simulink model "assignment_port_complex_test"  (Simulink 8.4)
settings: Solver=VariableStepDiscrete  StartTime=0.0  StopTime=0  MaxStep=1  RelTol=1e-3
settings Model: Creator=arnaud  LastModifiedBy=arnaud
settings DataIOCC: ExternalInput=xin  LoadExternalInput=on  SaveFormat=Structure  SignalLoggingSaveFormat=Dataset
settings OptimizationCC: ExpressionDepthLimit=128
settings DebuggingCC: UnderspecifiedInitializationDetection=Simplified  MergeDetectMultiDrivingBlocksExec=error  FcnCallInpInsideContextMsg=EnableAllAsError  StateNameClashWarn=none
settings GRTTargetCC: CombineOutputUpdateFcns=on  GRTInterface=off

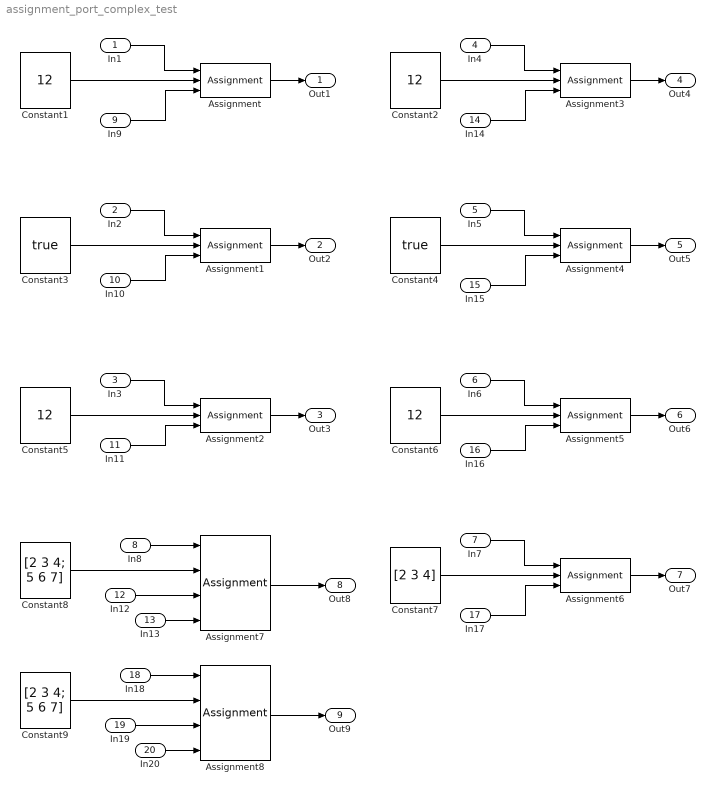
== system assignment_port_complex_test ==
  In1 : Inport  PortDimensions=[2 3]
      settings: SignalType=complex
  In2 : Inport  Port=2  OutDataTypeStr=boolean  PortDimensions=[2 3]
  In3 : Inport  Port=3  OutDataTypeStr=int32  PortDimensions=[2 3]
      settings: SignalType=complex
  In4 : Inport  Port=4  PortDimensions=3
      settings: SignalType=complex
  In5 : Inport  Port=5  OutDataTypeStr=boolean  PortDimensions=3
  In6 : Inport  Port=6  OutDataTypeStr=int32  PortDimensions=3
      settings: SignalType=complex
  In7 : Inport  Port=7  OutDataTypeStr=int32  PortDimensions=3
      settings: SignalType=complex
  In8 : Inport  Port=8  OutDataTypeStr=int32  PortDimensions=[2 3]
      settings: SignalType=complex
  In9 : Inport  Port=9  PortDimensions=2
  In10 : Inport  Port=10  OutDataTypeStr=int32
  In11 : Inport  Port=11  OutDataTypeStr=int32
  In12 : Inport  Port=12
  In13 : Inport  Port=13
  In14 : Inport  Port=14  PortDimensions=2
  In15 : Inport  Port=15
  In16 : Inport  Port=16
  In17 : Inport  Port=17
  In18 : Inport  Port=18  OutDataTypeStr=int32  PortDimensions=[2 3]
      settings: SignalType=complex
  In19 : Inport  Port=19
  In20 : Inport  Port=20
  Assignment : Assignment  NumberOfDimensions=2  DiagnosticForDimensions=Warning  IndexOptions=Index vector (port),Index vector (dialog)  Indices=[1 2],2  OutputSizes=1,1
  Assignment1 : Assignment  NumberOfDimensions=2  DiagnosticForDimensions=Warning  IndexOptions=Index vector (dialog),Index vector (port)  Indices=1,2  OutputSizes=1,1
  Assignment2 : Assignment  NumberOfDimensions=2  IndexMode=Zero-based  DiagnosticForDimensions=Warning  IndexOptions=Assign all,Index vector (port)  Indices=1,1  OutputSizes=1,1
  Assignment3 : Assignment  DiagnosticForDimensions=Warning  IndexOptions=Index vector (port)  Indices=[1 2]
  Assignment4 : Assignment  IndexMode=Zero-based  DiagnosticForDimensions=Warning  IndexOptions=Index vector (port)  Indices=2
  Assignment5 : Assignment  DiagnosticForDimensions=Warning  IndexOptions=Index vector (port)
  Assignment6 : Assignment  DiagnosticForDimensions=Warning  IndexOptions=Starting index (port)
  Assignment7 : Assignment  NumberOfDimensions=2  DiagnosticForDimensions=Warning  IndexOptions=Index vector (port),Index vector (port)  Indices=1,2  OutputSizes=1,1
  Assignment8 : Assignment  NumberOfDimensions=2  DiagnosticForDimensions=Warning  IndexOptions=Index vector (port),Starting index (port)  Indices=1,2  OutputSizes=1,1
  Constant1 : Constant  Value=12
  Constant2 : Constant  Value=12
  Constant3 : Constant  Value=true
  Constant4 : Constant  Value=true
  Constant5 : Constant  Value=12  OutDataTypeStr=int32
  Constant6 : Constant  Value=12  OutDataTypeStr=int32
  Constant7 : Constant  Value=[2 3 4]  OutDataTypeStr=int32
  Constant8 : Constant  Value=[2 3 4; 5 6 7]  OutDataTypeStr=int32
  Constant9 : Constant  Value=[2 3 4; 5 6 7]  OutDataTypeStr=int32
  Out1 : Outport
  Out2 : Outport  Port=2
  Out3 : Outport  Port=3
  Out4 : Outport  Port=4
  Out5 : Outport  Port=5
  Out6 : Outport  Port=6
  Out7 : Outport  Port=7
  Out8 : Outport  Port=8
  Out9 : Outport  Port=9
  wires:
  Assignment/1 -> Out1/1
  In1/1 -> Assignment/1
  Constant1/1 -> Assignment/2
  Assignment1/1 -> Out2/1
  In2/1 -> Assignment1/1
  Constant3/1 -> Assignment1/2
  Assignment2/1 -> Out3/1
  In3/1 -> Assignment2/1
  Constant5/1 -> Assignment2/2
  Assignment3/1 -> Out4/1
  In4/1 -> Assignment3/1
  Constant2/1 -> Assignment3/2
  Assignment4/1 -> Out5/1
  In5/1 -> Assignment4/1
  Constant4/1 -> Assignment4/2
  Assignment5/1 -> Out6/1
  In6/1 -> Assignment5/1
  Constant6/1 -> Assignment5/2
  Assignment6/1 -> Out7/1
  In7/1 -> Assignment6/1
  Constant7/1 -> Assignment6/2
  Assignment7/1 -> Out8/1
  In8/1 -> Assignment7/1
  Constant8/1 -> Assignment7/2
  In9/1 -> Assignment/3
  In10/1 -> Assignment1/3
  In11/1 -> Assignment2/3
  In12/1 -> Assignment7/3
  In13/1 -> Assignment7/4
  In14/1 -> Assignment3/3
  In15/1 -> Assignment4/3
  In16/1 -> Assignment5/3
  In17/1 -> Assignment6/3
  Assignment8/1 -> Out9/1
  In18/1 -> Assignment8/1
  Constant9/1 -> Assignment8/2
  In19/1 -> Assignment8/3
  In20/1 -> Assignment8/4
